simulink model "cart-pole-simu"  (R2017b)
settings: Solver=VariableStepAuto  StartTime=0.0  StopTime=10.0  RelTol=1e-3
settings Model: Creator=root  LastModifiedBy=root

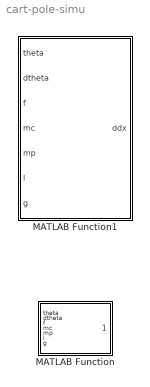
== system cart-pole-simu ==
  MATLAB Function : MATLAB Function  TreatAsAtomicUnit=on
  MATLAB Function1 : MATLAB Function  TreatAsAtomicUnit=on

== matlab function cart-pole-simu/MATLAB Function1 ==
  data: theta input; ddx output; dtheta input; f input; mc input; mp input; l input; g input
function ddx = ddx(theta, dtheta, f, mc, mp, l, g)

item1 = mc + mp * sin(theta).^2;
item2 = mp * sin(theta) * (l * dtheta^.2 + g * cos(theta));
ddx = 1/item1 * (f + item2);

end

== matlab function cart-pole-simu/MATLAB Function ==
  data: theta input; ddtheta output; dtheta input; f input; mc input; mp input; l input; g input
function ddtheta = ddtheta(theta, dtheta, f, mc, mp, l, g)

item1 = l * (mc + mp * sin(theta)^2);
item2 = mp * l * dtheta^.2 * cos(theta) * sin(theta);
item3 = (mc + mp) * g * sin(theta);

ddtheta = 1/item1 * (-f*cos(theta) - item2 - item3 );

end
